simulink model "Secondary"  (R2016b)
settings: Solver=FixedStepAuto  StartTime=0.0  StopTime=1000  RelTol=1e-3  EnableMultiTasking=on
libraries: dspsrcs4 x3, dspvision x2, dspsnks4 x1, simulink x1, dspadpt3 x1, audiosources x1
settings Model: Creator=xiezh  LastModifiedBy=xiezh
settings SolverCC: EnableConcurrentExecution=on
settings DataIOCC: SaveFormat=StructureWithTime
settings OptimizationCC: BlockReduction=off  OptimizeBlockIOStorage=off  BufferReuse=off  GlobalBufferReuse=off  ExpressionFolding=off  LocalBlockOutputs=off
settings HardwareCC: ProdBitPerPointer=32  ProdBitPerSizeT=32  ProdBitPerPtrDiffT=32  ProdLargestAtomicFloat=None  ProdWordSize=32  ProdLongLongMode=on  ProdHWDeviceType=Generic->32-bit x86 compatible
settings RTWCC: SystemTargetFile=slrt.tlc  TemplateMakefile=slrt_default_tmf  Description=Simulink Real-Time  RTWCompilerOptimization=on

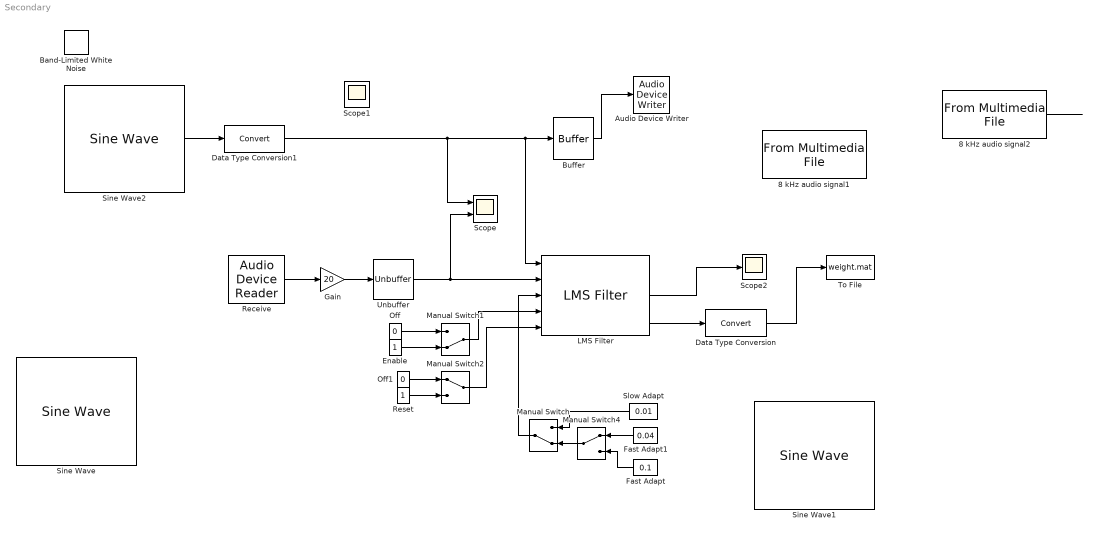
== system Secondary ==
  8 kHz audio signal1 : dspvision/From Multimedia File  inputFilename=C:\Users\xiezh\Documents\Signal&System\project\WN8.wav  loop=on  numPlays=inf  outputStreams=Audio only  videoDataType=single  audioDataType=single  inheritSampleTime=on  userDefinedSampleTime=1/8000  noAudioOutput=off  isIntensityVideo=off  fourcc=RGB  colorVideoFormat=Separate color signals  outputEOF=off  dataOrg=Column-major  audioFrameSize=32  computeAudioFrameSize=off  outSamplingMode=Sample based
  8 kHz audio signal2 : dspvision/From Multimedia File  inputFilename=C:\Users\xiezh\Documents\Signal&System\project\1_3white.wav  loop=on  numPlays=inf  outputStreams=Audio only  videoDataType=single  audioDataType=single  inheritSampleTime=off  userDefinedSampleTime=1/250  noAudioOutput=off  isIntensityVideo=off  fourcc=RGB  colorVideoFormat=Separate color signals  outputEOF=off  dataOrg=Column-major  audioFrameSize=32  computeAudioFrameSize=off  outSamplingMode=Sample based
  Audio Device Writer : dspsnks4/Audio Device Writer  Driver=ASIO  Device=ASIO4ALL v2  InheritSampleRate=on  SampleRate=8000  BitDepth=32-bit float  BufferSize=4096  NumBuffers=10  DefaultOutputChannelMapping=on  OutputChannelMapping=1:2  OutputNumUnderrunSamples=off  DriverIdx=3  DeviceWarnFlag=''
  Band-Limited White Noise : simulink/Sources/Band-Limited White Noise  Cov=[0.1]  Ts=1/8000  seed=[23341]
  Buffer : Buffer  N=32  TreatMby1Signals=One channel  OutputFrames=off
  Data Type Conversion : DataTypeConversion
  Data Type Conversion1 : DataTypeConversion
  Enable : Constant  OutDataTypeStr=boolean
  Fast Adapt : Constant  Value=0.1  OutDataTypeStr=single
  Fast Adapt1 : Constant  Value=0.04  OutDataTypeStr=single
  Gain : Gain  Gain=20
  LMS Filter : dspadpt3/LMS Filter  Algo=Normalized LMS  L=100  stepflag=Input port  mu=0  leakage=1  ic=[0]  Adapt=on  resetflag=Non-zero sample  weights=on  secondCoeffMode=User-defined  secondCoeffWordLength=2  secondCoeffFracLength=15  accum2Mode=User-defined  accum2FracLength=20  prodOutput2Mode=User-defined  prodOutput2FracLength=20  prodOutput3Mode=User-defined  prodOutput3FracLength=20  prodOutput4Mode=User-defined  prodOutput4FracLength=20  quotientMode=User-defined  quotientFracLength=20  roundingMode=Floor  overflowMode=off  addnparflag=off
  Manual Switch : ManualSwitch  CurrentSetting=0
  Manual Switch1 : ManualSwitch  CurrentSetting=0
  Manual Switch2 : ManualSwitch
  Manual Switch4 : ManualSwitch
  Off : Constant  Value=0  OutDataTypeStr=boolean
  Off1 : Constant  Value=0  OutDataTypeStr=boolean
  "Receive " : audiosources/Audio Device Reader  Driver=DirectSound  Device=Default  SampleRate=8000  NumChannels=1  SamplesPerFrame=32  BitDepth=32-bit float  NumBuffers=10  DefaultInputChannelMapping=on  InputChannelMapping=1:2  OutputNumOverrunSamples=off  OutputDataType=single  DriverIdx=1  DeviceWarnFlag=麦克风 (2- USB Audio Device)
  Reset : Constant  OutDataTypeStr=boolean
  Scope : Scope  NumInputPorts=2
  Scope2 : Scope
  Sine Wave : dspsrcs4/Sine Wave  Amplitude=[.1 .2 .5 -.7 .9 .3 -.9 .5 -.3]  Frequency=[3000 2000 2754 3237 2931 3211 2929 2155 2123]  Phase=[0 1 2 0 0 -2 2.3 5 5]  SampleMode=Discrete  OutComplex=Real  CompMethod=Trigonometric fcn  TableSize=Speed  SampleTime=1/8000  SamplesPerFrame=1  ResetState=Restart at time zero  OutputFrames=off  dataType=single  wordLen=16  udDataType=sfix(16)  fracBitsMode=Best precision  numFracBits=15  OutDataTypeStr=single  LastOutDataTypeStr=single
  Sine Wave1 : dspsrcs4/Sine Wave  Amplitude=[1]  Frequency=[2000]  Phase=[0]  SampleMode=Discrete  OutComplex=Real  CompMethod=Trigonometric fcn  TableSize=Speed  SampleTime=1/8000  SamplesPerFrame=1  ResetState=Restart at time zero  OutputFrames=off  dataType=single  wordLen=16  udDataType=sfix(16)  fracBitsMode=Best precision  numFracBits=15  OutDataTypeStr=single  LastOutDataTypeStr=single
  Sine Wave2 : dspsrcs4/Sine Wave  Amplitude=[1]  Frequency=[100]  Phase=[0]  SampleMode=Discrete  OutComplex=Real  CompMethod=Trigonometric fcn  TableSize=Speed  SampleTime=1/8000  SamplesPerFrame=1  ResetState=Restart at time zero  OutputFrames=off  dataType=single  wordLen=16  udDataType=sfix(16)  fracBitsMode=Best precision  numFracBits=15  OutDataTypeStr=single  LastOutDataTypeStr=single
  Slow Adapt : Constant  Value=0.01  OutDataTypeStr=single
  To File : ToFile  Filename=weight.mat
  Unbuffer : Unbuffer  SampleBasedProcessing=Same as frame based
  Scope1 : Scope
  wires:
  Off/1 -> Manual Switch1/1
  Enable/1 -> Manual Switch1/2
  Off1/1 -> Manual Switch2/1
  Reset/1 -> Manual Switch2/2
  Manual Switch2/1 -> LMS Filter/5
  Manual Switch1/1 -> LMS Filter/4
  Slow Adapt/1 -> Manual Switch/1
  Manual Switch4/1 -> Manual Switch/2
  Fast Adapt1/1 -> Manual Switch4/1
  Fast Adapt/1 -> Manual Switch4/2
  Manual Switch/1 -> LMS Filter/3
  LMS Filter/3 -> Data Type Conversion/1
  Data Type Conversion/1 -> To File/1
  "Receive "/1 -> Gain/1
  LMS Filter/2 -> Scope2/1
  Buffer/1 -> Audio Device Writer/1
  Gain/1 -> Unbuffer/1
  8 kHz audio signal2/1 -> ?
  Unbuffer/1 -> LMS Filter/2, Scope/2
  Sine Wave2/1 -> Data Type Conversion1/1
  Data Type Conversion1/1 -> Scope/1, LMS Filter/1, Buffer/1
